simulink model "cic_strukturen3"  (Simulink 7.8)
settings: Solver=ode45  StartTime=0.0  StopTime=10.0  RelTol=1e-3
values from neighbouring files (symbols this model uses):
  R = 4    [CFIR_1.m]    (also in cic_dezim1.m = 10; cic_dezim1_.m = ',num2str(R),'; cic_dezim2.m = 10)
libraries: dspsigops x4
settings Model: Creator=svenhoffmann  LastModifiedBy=josef  ExtModeAutoUpdateStatusClock=off
settings OptimizationCC: InlineInvariantSignals=on  InitFltsAndDblsToZero=on
settings DebuggingCC: SaveWithParameterizedLinksMsg=none  SignalResolutionControl=TryResolveAllWithWarning  MultiTaskDSMMsg=warning  MultiTaskCondExecSysMsg=none  StrictBusMsg=None
settings RTWCC: IncludeERTFirstTime=on
settings GRTTargetCC: TargetFcnLib=ansi_tfl_tmw.mat

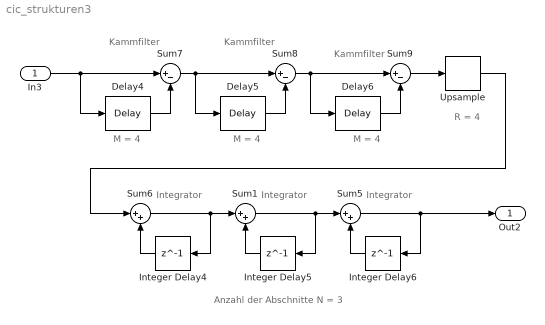
== system cic_strukturen3 ==
  note: R = 4
  note: Anzahl der Abschnitte N = 3
  note: M = 4
  note: Kammfilter
  note: M = 4
  note: M = 4
  note: Kammfilter
  note: Kammfilter
  note: Integrator
  note: Integrator
  note: Integrator
  In3 : Inport
  Delay4 : dspsigops/Delay  InputProcessing=Inherited (this choice will be removed - see release notes)  dly_unit=Samples  delay=M  ic_detail=off  dif_ic_for_ch=off  dif_ic_for_dly=off  ic=0  reset_popup=None
  Delay5 : dspsigops/Delay  InputProcessing=Inherited (this choice will be removed - see release notes)  dly_unit=Samples  delay=M  ic_detail=off  dif_ic_for_ch=off  dif_ic_for_dly=off  ic=0  reset_popup=None
  Delay6 : dspsigops/Delay  InputProcessing=Inherited (this choice will be removed - see release notes)  dly_unit=Samples  delay=M  ic_detail=off  dif_ic_for_ch=off  dif_ic_for_dly=off  ic=0  reset_popup=None
  Integer Delay4 : Delay  DelayLength=1  InputProcessing=Inherited
  Integer Delay5 : Delay  DelayLength=1  InputProcessing=Inherited
  Integer Delay6 : Delay  DelayLength=1  InputProcessing=Inherited
  Sum1 : Sum  Inputs=|++
  Sum5 : Sum  Inputs=|++
  Sum6 : Sum  Inputs=|++
  Sum7 : Sum  Inputs=|+-
  Sum8 : Sum  Inputs=|+-
  Sum9 : Sum  Inputs=|+-
  Upsample : dspsigops/Upsample  N=R  phase=0  InputProcessing=Inherited (this choice will be removed - see release notes)  RateOptions=Allow multirate processing  ic=0  mode=Unused parameter value
  Out2 : Outport
  wires:
  In3/1 -> Sum7/1, Delay4/1
  Delay4/1 -> Sum7/2
  Sum9/1 -> Upsample/1
  Delay5/1 -> Sum8/2
  Sum7/1 -> Delay5/1, Sum8/1
  Delay6/1 -> Sum9/2
  Sum8/1 -> Sum9/1, Delay6/1
  Sum6/1 -> Sum1/1, Integer Delay4/1
  Integer Delay4/1 -> Sum6/2
  Sum1/1 -> Sum5/1, Integer Delay5/1
  Integer Delay5/1 -> Sum1/2
  Sum5/1 -> Integer Delay6/1, Out2/1
  Integer Delay6/1 -> Sum5/2
  Upsample/1 -> Sum6/1
